simulink model "consensus_dead"  (R2024b)
settings: Solver=FixedStepAuto  StartTime=0.0  StopTime=Tf  FixedStep=dt  RelTol=1e-3
values from neighbouring files (symbols this model uses):
  A_an = ss_An.A    [red_consensus.m]    (also in red_consensus_2D.m; rendez_vous.m; squared_formation.m; triangular_formation.m)
  alpha = binvar(nt,nr)    [main_red_based_TA.m]    (also in motivating_ex_four.m = 25; old_red_based_TA.m = binvar(nt*nr,1); red_consensus.m = 50; red_consensus_2D.m = 50)
  B = eye(n)    [red_consensus.m]    (also in red_consensus_2D.m = eye(2*n); rendez_vous.m = eye(2*n_t3); squared_formation.m = eye(2*n_t2); squared_formation_dec.m = eye(2*n_t2))
  B_an = ss_An.B    [red_consensus.m]    (also in red_consensus_2D.m; rendez_vous.m; squared_formation.m; triangular_formation.m)
  C = 50    [old_red_based_TA.m]    (also in red_consensus.m = L; red_consensus_2D.m = blkdiag(L,L); rendez_vous.m = blkdiag(Lt3,Lt3); squared_formation.m = blkdiag(Lt2,Lt2))
  C_an = ss_An.C    [red_consensus.m]    (also in red_consensus_2D.m; rendez_vous.m; squared_formation.m; triangular_formation.m)
  C_opt = 1    [motivating_ex_four.m]    (also in red_consensus.m; red_consensus_2D.m = eye(2); rendez_vous.m = eye(2); squared_formation.m = eye(2))
  D_an = ss_An.D    [red_consensus.m]    (also in red_consensus_2D.m; rendez_vous.m; squared_formation.m; triangular_formation.m)
  delta = binvar(nr,1)    [main_red_based_TA.m]    (also in red_consensus.m = [2 1 0 -1 -2 -1  1]'; red_consensus_2D.m = [delta_x;delta_y]; rendez_vous.m = [delta_x_t3;delta_y_t3]; squared_formation.m = [delta_x_t2;delta_y_t2])
  f = 0.2    [consensus.m]    (also in consensus_sat.m; red_consensus.m = 1; red_consensus_2D.m; rendez_vous.m)
  sig_vec = ones(num,1)    [rendez_vous.m]    (also in squared_formation.m; squared_formation_dec.m; triangular_formation.m)
  th = 0.05    [motivating_ex_four.m]    (also in red_consensus.m; red_consensus_2D.m; triangular_formation.m)
  u_max = [1,0.5,1,0.4,1.5,0.5,1]'    [red_consensus.m]    (also in red_consensus_2D.m = [u_max_x;u_max_y]; rendez_vous.m = [u_max_x(cc{idx3});u_max_y(cc{idx3})]; squared_formation.m = [u_max_x(cc{idx2});u_max_y(cc{idx2})]; squared_formation_dec.m = [u_max_x(cc{idx2});u_max_y(cc{idx2})])
  W_an0 = dcgain(W_an)    [red_consensus.m]    (also in red_consensus_2D.m; rendez_vous.m; squared_formation.m; triangular_formation.m)
  x0 = zeros(na,1)    [main_red_based_TA.m]    (also in red_consensus.m = zeros(n,1); red_consensus_2D.m = zeros(n,1); rendez_vous.m = x0_cc3; squared_formation.m = x0_cc2)
  x_an0 = zeros(max(size(A_an)),1)    [red_consensus.m]    (also in red_consensus_2D.m; rendez_vous.m; squared_formation.m; squared_formation_dec.m = zeros(max(size(A_an_n2)),1))
  x_opt0 = 0    [red_consensus.m]    (also in red_consensus_2D.m = zeros(2,1); rendez_vous.m = zeros(2,1); squared_formation.m = zeros(2,1); squared_formation_dec.m = zeros(2,1))
  y0 = zeros(na,1)    [main_red_based_TA.m]    (also in red_consensus_2D.m = zeros(n,1); rendez_vous.m = y0_cc3; squared_formation.m = y0_cc2; triangular_formation.m = y0_cc1)
settings Model: Creator=lorenzo  LastModifiedBy=lorenzo
settings SolverCC: ZeroCrossControl=DisableAll
settings DebuggingCC: IgnoredZcDiagnostic=none
settings RTWCC: GPUComputeCapability=3.5

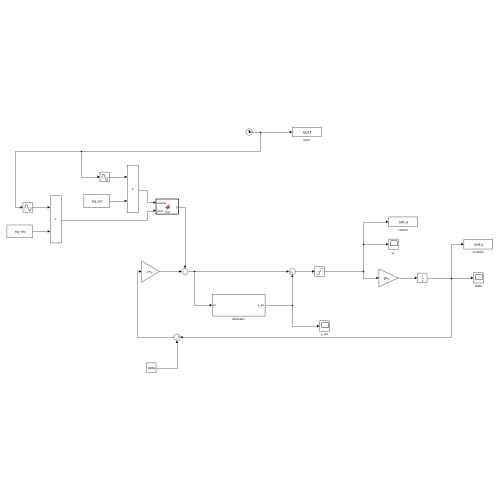
[thumbnail: Simulink's stored preview of the top-level diagram]
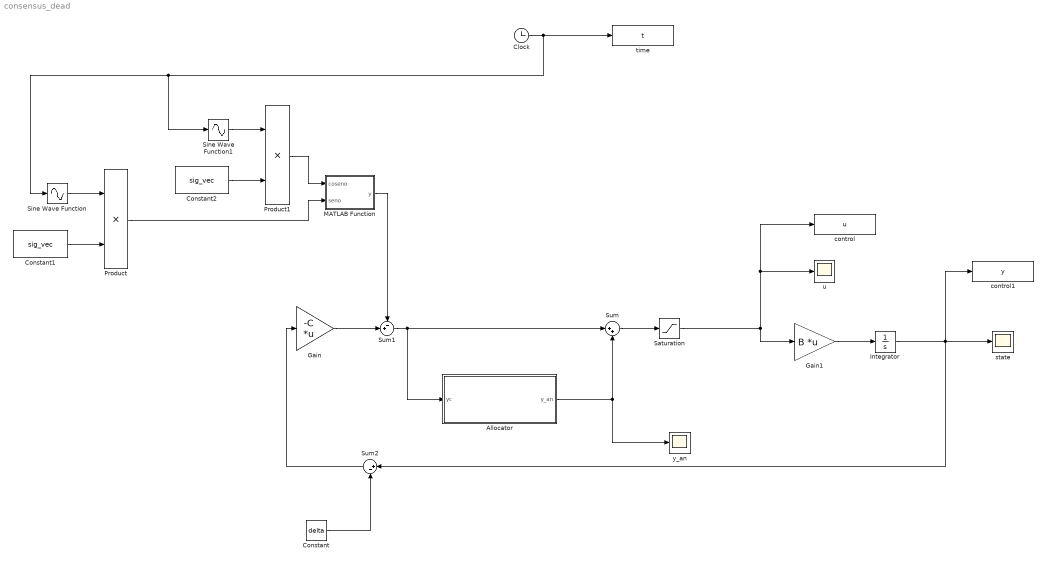
== system consensus_dead ==
  Allocator : Subsystem
  Clock : Clock
  Constant : Constant  Value=delta  VectorParams1D=off
  Constant1 : Constant  Value=sig_vec  VectorParams1D=off
  Constant2 : Constant  Value=sig_vec  VectorParams1D=off
  Gain : Gain  Gain=-C  Multiplication=Matrix(K*u)
  Gain1 : Gain  Gain=B  Multiplication=Matrix(K*u)
  Integrator : Integrator  InitialCondition=[x0;y0]
  MATLAB Function : MATLAB Function  TreatAsAtomicUnit=on
  Product : Product
  Product1 : Product
  Saturation : Saturate  UpperLimit=u_max  LowerLimit=-u_max
  Sine Wave Function : Sin  TimeSource=Use external signal  Frequency=f  SampleTime=0
  Sine Wave Function1 : Sin  TimeSource=Use external signal  Frequency=f  Phase=pi/2  SampleTime=0
  Sum : Sum  Inputs=|++
  Sum1 : Sum  Inputs=-+|  InputSameDT=on
  Sum2 : Sum  Inputs=|+-
  control : ToWorkspace  VariableName=u  SampleTime=-1
  control1 : ToWorkspace  VariableName=y  SampleTime=-1
  state : Scope
  time : ToWorkspace  VariableName=t  SampleTime=-1
  u : Scope
  y_an : Scope
  wires:
  Sum/1 -> Saturation/1
  Gain1/1 -> Integrator/1
  Saturation/1 -> Gain1/1, control/1, u/1
  Allocator/1(y_an) -> Sum/2, y_an/1
  Gain/1 -> Sum1/2
  Sum1/1 -> Allocator/1(yc), Sum/1
  Constant/1 -> Sum2/2
  Integrator/1 -> Sum2/1, control1/1, state/1
  Sum2/1 -> Gain/1
  Constant1/1 -> Product/2
  Sine Wave Function/1 -> Product/1
  Clock/1 -> Sine Wave Function1/1, Sine Wave Function/1, time/1
  Constant2/1 -> Product1/2
  Sine Wave Function1/1 -> Product1/1
  Product1/1 -> MATLAB Function/1(coseno)
  MATLAB Function/1(y) -> Sum1/1
  Product/1 -> MATLAB Function/2(seno)

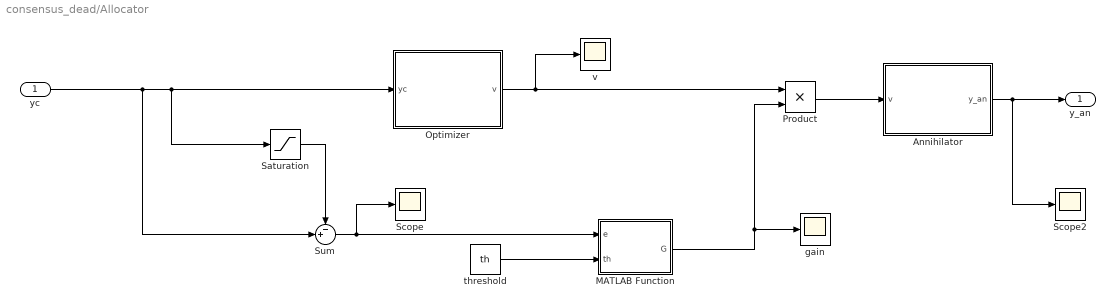
== system consensus_dead/Allocator ==
  yc : Inport
  Annihilator : Subsystem
  MATLAB Function : MATLAB Function  TreatAsAtomicUnit=on
  Optimizer : Subsystem
  Product : Product
  Saturation : Saturate  UpperLimit=u_max  LowerLimit=-u_max
  Scope : Scope
  Scope2 : Scope
  Sum : Sum  Inputs=-+|
  gain : Scope
  threshold : Constant  Value=th
  v : Scope
  y_an : Outport
  wires:
  threshold/1 -> MATLAB Function/2(th)
  yc/1 -> Sum/2, Saturation/1, Optimizer/1(yc)
  Product/1 -> Annihilator/1(v)
  Annihilator/1(y_an) -> Scope2/1, y_an/1
  MATLAB Function/1(G) -> Product/2, gain/1
  Optimizer/1(v) -> v/1, Product/1
  Saturation/1 -> Sum/1
  Sum/1 -> MATLAB Function/1(e), Scope/1

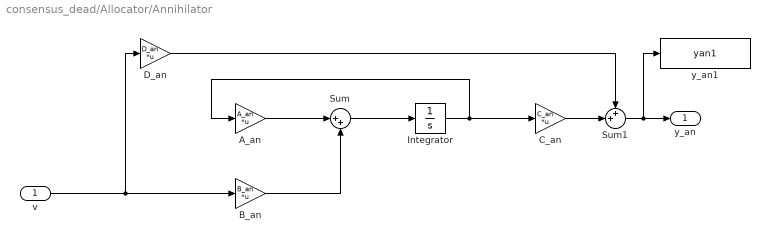
== system consensus_dead/Allocator/Annihilator ==
  v : Inport
  A_an : Gain  Gain=A_an  Multiplication=Matrix(K*u) (u vector)
  B_an : Gain  Gain=B_an  Multiplication=Matrix(K*u) (u vector)
  C_an : Gain  Gain=C_an  Multiplication=Matrix(K*u) (u vector)
  D_an : Gain  Gain=D_an  Multiplication=Matrix(K*u) (u vector)
  Integrator : Integrator  InitialCondition=x_an0
  Sum : Sum  Inputs=|++
  Sum1 : Sum  Inputs=++|
  y_an1 : ToWorkspace  VariableName=yan1  SampleTime=-1
  y_an : Outport
  wires:
  Integrator/1 -> C_an/1, A_an/1
  B_an/1 -> Sum/2
  A_an/1 -> Sum/1
  Sum/1 -> Integrator/1
  C_an/1 -> Sum1/2
  D_an/1 -> Sum1/1
  Sum1/1 -> y_an1/1, y_an/1
  v/1 -> B_an/1, D_an/1

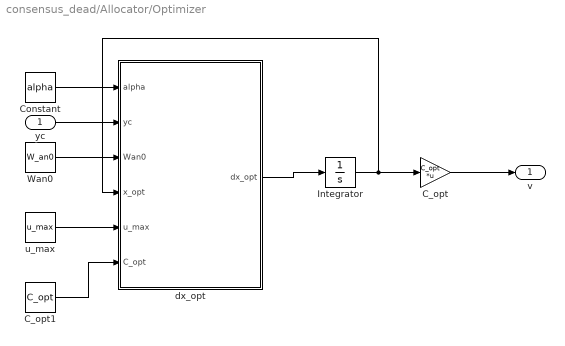
== system consensus_dead/Allocator/Optimizer ==
  yc : Inport
  C_opt : Gain  Gain=C_opt  Multiplication=Matrix(K*u) (u vector)
  C_opt1 : Constant  Value=C_opt
  Constant : Constant  Value=alpha
  Integrator : Integrator  InitialCondition=x_opt0
  Wan0 : Constant  Value=W_an0  VectorParams1D=off
  dx_opt : MATLAB Function  TreatAsAtomicUnit=on
  u_max : Constant  Value=u_max
  v : Outport
  wires:
  Integrator/1 -> C_opt/1, dx_opt/4(x_opt)
  dx_opt/1(dx_opt) -> Integrator/1
  C_opt/1 -> v/1
  Constant/1 -> dx_opt/1(alpha)
  yc/1 -> dx_opt/2(yc)
  Wan0/1 -> dx_opt/3(Wan0)
  u_max/1 -> dx_opt/5(u_max)
  C_opt1/1 -> dx_opt/6(C_opt)

== matlab function consensus_dead/Allocator/MATLAB Function ==
  data: e input; G output; th input
function G = fcn(e,th)
norm(e);
eps = th/2;

G=1;

% if ( norm(e) < th-eps )
%     G = 0;
% end
% if ( norm(e) > th )
%     G = 1;
% end
% if ( norm(e) <= th && norm(e) >= th-eps )
%     G = -2*((norm(e)-(th-eps))/eps)^3+3*((norm(e)-(th-eps))/eps)^2;
% end

== matlab function consensus_dead/MATLAB Function ==
  data: coseno input; y output; seno input
function y = fcn(coseno, seno)

y = [coseno;seno];

== matlab function consensus_dead/Allocator/Optimizer/dx_opt ==
  data: dx_opt output; alpha input; yc input; Wan0 input; x_opt input; u_max input; C_opt input
function dx_opt = opt_dyn(alpha,yc,Wan0,x_opt,u_max,C_opt)

% u1_max = u_max(1);
% u2_max = u_max(2);
% u3_max = u_max(3);
% u4_max = u_max(4);
% u5_max = u_max(5);
% u6_max = u_max(6);
% u7_max = u_max(7);
% 
% u11_max = u_max(8);
% u22_max = u_max(9);
% u33_max = u_max(10);
% u44_max = u_max(11);
% u55_max = u_max(12);
% u66_max = u_max(13);
% u77_max = u_max(14);

dim = max(size(u_max));

ss_u = yc+Wan0*C_opt*x_opt;

ss_sat = ss_u;

for i=1:dim
    if ( abs(ss_u(i))>= u_max(i) )
        ss_sat(i) = sign(ss_u(i))*u_max(i);
    end
end

% if ( abs(ss_u(1))>=u1_max )
%     ss_sat(1) = sign(ss_u(1))*u1_max;
% end
% if ( abs(ss_u(2))>=u2_max )
%     ss_sat(2) = sign(ss_u(2))*u2_max;
% end
% if ( abs(ss_u(3))>=u3_max )
%     ss_sat(3) = sign(ss_u(3))*u3_max;
% end
% if ( abs(ss_u(4))>=u4_max )
%     ss_sat(4) = sign(ss_u(4))*u4_max;
% end
% if ( abs(ss_u(5))>=u5_max )
%     ss_sat(5) = sign(ss_u(5))*u5_max;
% end
% if ( abs(ss_u(6))>=u6_max )
%     ss_sat(6) = sign(ss_u(6))*u6_max;
% end
% if ( abs(ss_u(7))>=u7_max )
%     ss_sat(7) = sign(ss_u(7))*u7_max;
% end
% 
% if ( abs(ss_u(8))>=u11_max )
%     ss_sat(8) = sign(ss_u(8))*u11_max;
% end
% if ( abs(ss_u(9))>=u22_max )
%     ss_sat(9) = sign(ss_u(9))*u22_max;
% end
% if ( abs(ss_u(10))>=u33_max )
%     ss_sat(10) = sign(ss_u(10))*u33_max;
% end
% if ( abs(ss_u(11))>=u44_max )
%     ss_sat(11) = sign(ss_u(11))*u44_max;
% end
% if ( abs(ss_u(12))>=u55_max )
%     ss_sat(12) = sign(ss_u(12))*u55_max;
% end
% if ( abs(ss_u(13))>=u66_max )
%     ss_sat(13) = sign(ss_u(13))*u66_max;
% end
% if ( abs(ss_u(14))>=u77_max )
%     ss_sat(14) = sign(ss_u(14))*u77_max;
% end

par_der = zeros(dim,dim);

for i =1:dim
    par_der(i,i) = dsat(ss_u(i),u_max(i),0.01);
end

% par_der = diag([dsat(ss_u(1),u1_max,0.01), ...
%                 dsat(ss_u(2),u2_max,0.01), ...
%                 dsat(ss_u(3),u3_max,0.01), ...
%                 dsat(ss_u(4),u4_max,0.01), ...
%                 dsat(ss_u(5),u5_max,0.01), ...
%                 dsat(ss_u(6),u6_max,0.01), ...
%                 dsat(ss_u(7),u7_max,0.01), ...
%                 dsat(ss_u(8),u11_max,0.01), ...
%                 dsat(ss_u(9),u22_max,0.01), ...
%                 dsat(ss_u(10),u33_max,0.01), ...
%                 dsat(ss_u(11),u44_max,0.01), ...
%                 dsat(ss_u(12),u55_max,0.01), ...
%                 dsat(ss_u(13),u66_max,0.01), ...
%                 dsat(ss_u(14),u77_max,0.01),]); 

grad = (ss_u-ss_sat)'*(Wan0*C_opt-par_der*Wan0*C_opt);

dx_opt = -alpha*grad';
